simulink model "interface_simmetis"  (Simulink 7.0)
settings: Solver=ode45  StartTime=0.0  StopTime=10.0  RelTol=1e-3
libraries: simulink x21
settings Model: Creator=JA132999  LastModifiedBy=artaud  ExtModeAutoUpdateStatusClock=off
settings DebuggingCC: SaveWithParameterizedLinksMsg=none  SignalResolutionControl=TryResolveAllWithWarning  MultiTaskDSMMsg=warning  MultiTaskCondExecSysMsg=none
settings RTWCC: IncludeERTFirstTime=on
settings GRTTargetCC: TargetFcnLib=ansi_tfl_tmw.mat

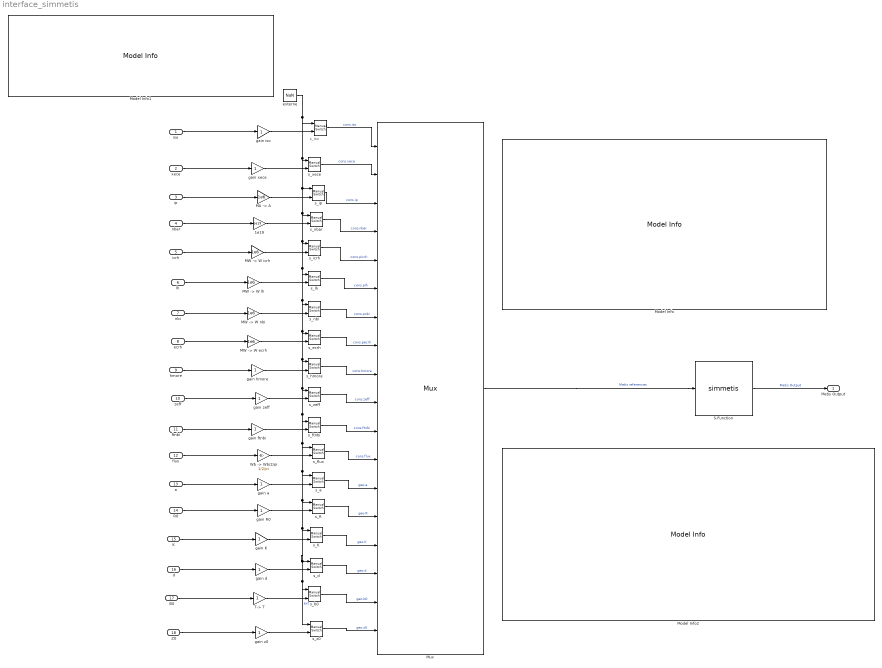
== system interface_simmetis ==
  note: s_iso
  iso : Inport  OutDataType=sfix(16)  OutScaling=2^0
  xece : Inport  Port=2  OutDataType=sfix(16)  OutScaling=2^0
  ip : Inport  Port=3  OutDataType=sfix(16)  OutScaling=2^0
  nbar : Inport  Port=4  OutDataType=sfix(16)  OutScaling=2^0
  icrh : Inport  Port=5  OutDataType=sfix(16)  OutScaling=2^0
  lh : Inport  Port=6  OutDataType=sfix(16)  OutScaling=2^0
  nbi : Inport  Port=7  OutDataType=sfix(16)  OutScaling=2^0
  ecrh : Inport  Port=8  OutDataType=sfix(16)  OutScaling=2^0
  hmore : Inport  Port=9  OutDataType=sfix(16)  OutScaling=2^0
  zeff : Inport  Port=10  OutDataType=sfix(16)  OutScaling=2^0
  ftnbi : Inport  Port=11  OutDataType=sfix(16)  OutScaling=2^0
  flux : Inport  Port=12  OutDataType=sfix(16)  OutScaling=2^0
  a : Inport  Port=13  OutDataType=sfix(16)  OutScaling=2^0
  R0 : Inport  Port=14  OutDataType=sfix(16)  OutScaling=2^0
  K : Inport  Port=15  OutDataType=sfix(16)  OutScaling=2^0
  d : Inport  Port=16  OutDataType=sfix(16)  OutScaling=2^0
  B0 : Inport  Port=17  OutDataType=sfix(16)  OutScaling=2^0
  Z0 : Inport  Port=18  OutDataType=sfix(16)  OutScaling=2^0
  " " : simulink/Signal Routing/Manual Switch  SystemSampleTime=-1  sw=1  action=0  varsize=off
  1e19 : Gain  Gain=1e19  ParameterDataType=sfix(16)  ParameterScaling=2^0  OutDataType=sfix(16)  OutScaling=2^0
  "MA -> A" : Gain  Gain=1e6  ParameterDataType=sfix(16)  ParameterScaling=2^0  OutDataType=sfix(16)  OutScaling=2^0
  "MW -> W ecrh" : Gain  Gain=1e6  ParameterDataType=sfix(16)  ParameterScaling=2^0  OutDataType=sfix(16)  OutScaling=2^0
  "MW -> W icrh" : Gain  Gain=1e6  ParameterDataType=sfix(16)  ParameterScaling=2^0  OutDataType=sfix(16)  OutScaling=2^0
  "MW -> W lh" : Gain  Gain=1e6  ParameterDataType=sfix(16)  ParameterScaling=2^0  OutDataType=sfix(16)  OutScaling=2^0
  "MW -> W nbi" : Gain  Gain=1e6  ParameterDataType=sfix(16)  ParameterScaling=2^0  OutDataType=sfix(16)  OutScaling=2^0
  Model Info : simulink/Model-Wide Utilities/Model Info  SystemSampleTime=-1  InitialBlockCM=None  BlockCM=None  Frame=on  DisplayStringWithTags=|  HorizontalTextAlignment=Center  LeftAlignmentValue=0.5  SourceBlockDiagram=interface_simmetis  TagMaxNumber=20
      | Interface_SimMetis : Library simmetis interface
      | %<Created>
      | %<ModifiedBy>
      | %<ModifiedDate>
      | %<ModifiedComment>
      | %<Description>
  Model Info1 : simulink/Model-Wide Utilities/Model Info  SystemSampleTime=-1  InitialBlockCM=None  BlockCM=None  Frame=on  DisplayStringWithTags=|  HorizontalTextAlignment=Center  LeftAlignmentValue=0.5  SourceBlockDiagram=interface_simmetis  TagMaxNumber=20
      | when an input is set to NaN, 
      | the correspondant reference value
      | is read from Metis file (or data) 
      | and linearely interpolate in time.
  Model Info2 : simulink/Model-Wide Utilities/Model Info  SystemSampleTime=-1  InitialBlockCM=None  BlockCM=None  Frame=on  DisplayStringWithTags=|  HorizontalTextAlignment=Left  LeftAlignmentValue=0.02  SourceBlockDiagram=interface_simmetis  TagMaxNumber=20
      | Simmetis parameters :
      | * Metis_file_name : used to parametring Metis in simmetis 
      | (if empty used z0dinput in workspace,
      |  that allow to tune simulation configuration form Metis interface)
      | * list_output : cell array of output names
      | * save_file : results filename (optionnel)
      | * verbose  : if = 1 turn on information writing
      | * input_option:  optionnal cell list of METIS option parameter used as input of the S-function   
      |   (example : {'npar0'})
  Mux : Mux  Tag=Metis refererences  Inputs=18
      settings: DisplayOption=signals
  S-Function : S-Function  FunctionName=simmetis  Parameters='',{},'',0
  T-> T : Gain  ParameterDataType=sfix(16)  ParameterScaling=2^0  OutDataType=sfix(16)  OutScaling=2^0
  "Wb -> Wb/2/pi" : Gain  Gain=1/2/pi  ParameterDataType=sfix(16)  ParameterScaling=2^0  OutDataType=sfix(16)  OutScaling=2^0
  externe : Constant  Value=NaN  OutDataType=sfix(16)  OutScaling=2^0
  gain K : Gain  ParameterDataType=sfix(16)  ParameterScaling=2^0  OutDataType=sfix(16)  OutScaling=2^0
  gain R0 : Gain  ParameterDataType=sfix(16)  ParameterScaling=2^0  OutDataType=sfix(16)  OutScaling=2^0
  gain a : Gain  ParameterDataType=sfix(16)  ParameterScaling=2^0  OutDataType=sfix(16)  OutScaling=2^0
  gain d : Gain  ParameterDataType=sfix(16)  ParameterScaling=2^0  OutDataType=sfix(16)  OutScaling=2^0
  gain ftnbi : Gain  ParameterDataType=sfix(16)  ParameterScaling=2^0  OutDataType=sfix(16)  OutScaling=2^0
  gain hmore : Gain  ParameterDataType=sfix(16)  ParameterScaling=2^0  OutDataType=sfix(16)  OutScaling=2^0
  gain iso : Gain  ParameterDataType=sfix(16)  ParameterScaling=2^0  OutDataType=sfix(16)  OutScaling=2^0
  gain xece : Gain  ParameterDataType=sfix(16)  ParameterScaling=2^0  OutDataType=sfix(16)  OutScaling=2^0
  gain z0 : Gain  ParameterDataType=sfix(16)  ParameterScaling=2^0  OutDataType=sfix(16)  OutScaling=2^0
  gain zeff : Gain  ParameterDataType=sfix(16)  ParameterScaling=2^0  OutDataType=sfix(16)  OutScaling=2^0
  s_K : simulink/Signal Routing/Manual Switch  SystemSampleTime=-1  sw=1  action=0  varsize=off
  s_R : simulink/Signal Routing/Manual Switch  SystemSampleTime=-1  sw=1  action=0  varsize=off
  s_a : simulink/Signal Routing/Manual Switch  SystemSampleTime=-1  sw=1  action=0  varsize=off
  s_b0 : simulink/Signal Routing/Manual Switch  SystemSampleTime=-1  sw=1  action=0  varsize=off
  s_d : simulink/Signal Routing/Manual Switch  SystemSampleTime=-1  sw=1  action=0  varsize=off
  s_ecrh : simulink/Signal Routing/Manual Switch  SystemSampleTime=-1  sw=1  action=0  varsize=off
  s_flux : simulink/Signal Routing/Manual Switch  SystemSampleTime=-1  sw=1  action=0  varsize=off
  s_ftnbi : simulink/Signal Routing/Manual Switch  SystemSampleTime=-1  sw=1  action=0  varsize=off
  s_hmore : simulink/Signal Routing/Manual Switch  SystemSampleTime=-1  sw=1  action=0  varsize=off
  s_icrh : simulink/Signal Routing/Manual Switch  SystemSampleTime=-1  sw=1  action=0  varsize=off
  s_ip : simulink/Signal Routing/Manual Switch  SystemSampleTime=-1  sw=1  action=0  varsize=off
  s_lh : simulink/Signal Routing/Manual Switch  SystemSampleTime=-1  sw=1  action=0  varsize=off
  s_nbar : simulink/Signal Routing/Manual Switch  SystemSampleTime=-1  sw=1  action=0  varsize=off
  s_nbi : simulink/Signal Routing/Manual Switch  SystemSampleTime=-1  sw=1  action=0  varsize=off
  s_xece : simulink/Signal Routing/Manual Switch  SystemSampleTime=-1  sw=1  action=0  varsize=off
  s_z0 : simulink/Signal Routing/Manual Switch  SystemSampleTime=-1  sw=1  action=0  varsize=off
  s_zeff : simulink/Signal Routing/Manual Switch  SystemSampleTime=-1  sw=1  action=0  varsize=off
  Metis Output : Outport  OutDataType=sfix(16)  OutScaling=2^0
  wires:
  S-Function/1 -> Metis Output/1  "Metis Output"
  Mux/1 -> S-Function/1  "Metis references"
  externe/1 -> " "/1, s_xece/1, s_ip/1, s_nbar/1, s_icrh/1, s_lh/1, s_nbi/1, s_ecrh/1, s_hmore/1, s_zeff/1, s_ftnbi/1, s_flux/1, s_a/1, s_R/1, s_K/1, s_d/1, s_b0/1, s_z0/1  "ext"
  " "/1 -> Mux/1  "cons.iso"
  iso/1 -> gain iso/1
  gain iso/1 -> " "/2
  s_xece/1 -> Mux/2  "cons.xece"
  xece/1 -> gain xece/1
  gain xece/1 -> s_xece/2
  ip/1 -> "MA -> A"/1
  "MA -> A"/1 -> s_ip/2
  s_ip/1 -> Mux/3  "cons.ip"
  nbar/1 -> 1e19/1
  1e19/1 -> s_nbar/2
  s_nbar/1 -> Mux/4  "cons.nbar"
  icrh/1 -> "MW -> W icrh"/1
  "MW -> W icrh"/1 -> s_icrh/2
  s_icrh/1 -> Mux/5  "cons.picrh"
  lh/1 -> "MW -> W lh"/1
  "MW -> W lh"/1 -> s_lh/2
  s_lh/1 -> Mux/6  "cons.plh"
  nbi/1 -> "MW -> W nbi"/1
  "MW -> W nbi"/1 -> s_nbi/2
  s_nbi/1 -> Mux/7  "cons.pnbi"
  ecrh/1 -> "MW -> W ecrh"/1
  "MW -> W ecrh"/1 -> s_ecrh/2
  s_ecrh/1 -> Mux/8  "cons.pecrh"
  hmore/1 -> gain hmore/1
  gain hmore/1 -> s_hmore/2
  s_hmore/1 -> Mux/9  "cons.hmore"
  zeff/1 -> gain zeff/1
  gain zeff/1 -> s_zeff/2
  s_zeff/1 -> Mux/10  "cons.zeff"
  ftnbi/1 -> gain ftnbi/1
  gain ftnbi/1 -> s_ftnbi/2
  s_ftnbi/1 -> Mux/11  "cons.ftnbi"
  flux/1 -> "Wb -> Wb/2/pi"/1
  "Wb -> Wb/2/pi"/1 -> s_flux/2
  s_flux/1 -> Mux/12  "cons.flux"
  a/1 -> gain a/1
  gain a/1 -> s_a/2
  B0/1 -> T-> T/1
  T-> T/1 -> s_b0/2
  s_a/1 -> Mux/13  "geo.a"
  R0/1 -> gain R0/1
  gain R0/1 -> s_R/2
  s_R/1 -> Mux/14  "geo.R"
  K/1 -> gain K/1
  gain K/1 -> s_K/2
  s_K/1 -> Mux/15  "geo.K"
  d/1 -> gain d/1
  gain d/1 -> s_d/2
  s_d/1 -> Mux/16  "geo.d"
  Z0/1 -> gain z0/1
  gain z0/1 -> s_z0/2
  s_b0/1 -> Mux/17  "geo.b0"
  s_z0/1 -> Mux/18  "geo.z0"
